simulink model "Stoppuhr"  (Simulink 4.00)
settings: Solver=FixedStepDiscrete  StartTime=0.0  StopTime=10000000000.  FixedStep=0.001  RelTol=1e-3
libraries: simulink3 x3
settings Model: BlockReductionOpt=off

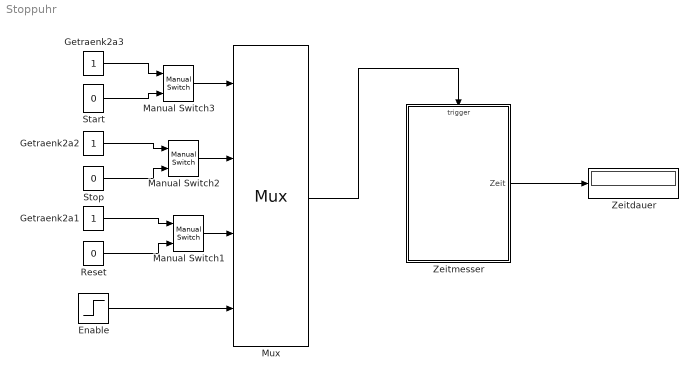
== system Stoppuhr ==
  Enable : Step  Time=0.1  Before=0  After=1  SampleTime=0
  Getraenk2a1 : Constant  Value=1
  Getraenk2a2 : Constant  Value=1
  Getraenk2a3 : Constant  Value=1
  Manual Switch1 : simulink3/Nonlinear/Manual Switch  sw=0  action=0
  Manual Switch2 : simulink3/Nonlinear/Manual Switch  sw=0  action=0
  Manual Switch3 : simulink3/Nonlinear/Manual Switch  sw=0  action=0
  Mux : Mux  Inputs=4
      settings: DisplayOption=none
  Reset : Constant  Value=0
  Start : Constant  Value=0
  Stop : Constant  Value=0
  Zeitdauer : Display
      settings: Format=short
  Zeitmesser : Stateflow chart  TreatAsAtomicUnit=on
      settings: RTWFcnNameOpts=Auto  RTWFileNameOpts=Auto
  wires:
  Mux/1 -> Zeitmesser/Trigger
  Getraenk2a2/1 -> Manual Switch2/1
  Getraenk2a3/1 -> Manual Switch3/1
  Manual Switch1/1 -> Mux/3
  Zeitmesser/1(Zeit) -> Zeitdauer/1
  Enable/1 -> Mux/4
  Manual Switch3/1 -> Mux/1
  Manual Switch2/1 -> Mux/2
  Stop/1 -> Manual Switch2/2
  Start/1 -> Manual Switch3/2
  Getraenk2a1/1 -> Manual Switch1/1
  Reset/1 -> Manual Switch1/2

== stateflow chart Zeitmesser ==
  state Ruhezustand/
    entry:Zeit=0;
  state Zeit_steht/
    entry: Zeit=Zeit+DT;
    exit:  DT=0;
  state Zeit_laeuft/
  (default) -> Ruhezustand
  Zeit_steht -> Ruhezustand : Reset
  Zeit_steht -> Zeit_laeuft : Start/ml('tic')
  Zeit_laeuft -> Zeit_steht : Stop/DT=ml('toc')
  Ruhezustand -> Zeit_laeuft : Start/ml('tic')
  data: Zeit output double; DT local double
  events: Start input EITHER_EDGE_EVENT; Stop input EITHER_EDGE_EVENT; Reset input EITHER_EDGE_EVENT; Enable input EITHER_EDGE_EVENT
